simulink model "gm_Watermarker_ref"  (R2022a)
settings: Solver=FixedStepDiscrete  StartTime=0.0  StopTime=256*256-1  RelTol=1e-3
libraries: hdlsllib x10, dspsrcs4 x4
Description:
  | Performs watermarking.
  | In:
  | - One channel of 8-bit image 256x256
  | - Watermark (64 bits)
  | Out:
  | - Watermarked image channel
settings Model: SimulationMode=accelerator  Creator=The MathWorks, Inc.  LastModifiedBy=Администратор
settings SolverCC: AlgebraicLoopSolver=TrustRegion
settings DataIOCC: ExternalInput=image_and_mes_t.getElement('pixel_in'),image_and_mes_t.getElement('mes_in')  LimitDataPoints=on  LoadExternalInput=on  SaveFormat=Structure  SaveTime=off  ReturnWorkspaceOutputs=off
settings OptimizationCC: BlockReduction=off  ConditionallyExecuteInputs=off  DefaultParameterBehavior=Inlined  InheritOutputTypeSmallerThanSingle=on  OptimizeBlockIOStorage=off  DenormalBehavior=FlushToZero
settings DebuggingCC: AlgebraicLoopMsg=error  UnderspecifiedInitializationDetection=Classic  MergeDetectMultiDrivingBlocksExec=none  SolverPrmCheckMsg=warning  InheritedTsInSrcMsg=none  SingleTaskRateTransMsg=error  ParameterPrecisionLossMsg=none  UnconnectedInputMsg=warning  UnconnectedOutputMsg=warning  UnconnectedLineMsg=warning  AllowSymbolicDim=off  SFUnexpectedBacktrackingDiag=warning  SFNoUnconditionalDefaultTransitionDiag=warning  SFExecutionAtInitializationDiag=none  SFMachineParentedDataDiag=warning  ArithmeticOperatorsInVariantConditions=warning
settings HardwareCC: ProdBitPerPointer=32  ProdBitPerSizeT=32  ProdBitPerPtrDiffT=32  ProdLargestAtomicFloat=None  ProdIntDivRoundTo=Undefined  ProdEndianess=Unspecified  ProdWordSize=32  ProdHWDeviceType=ASIC/FPGA->ASIC/FPGA  TargetBitPerPointer=64  TargetBitPerSizeT=64  TargetBitPerPtrDiffT=64  TargetLongLongMode=on  TargetIntDivRoundTo=Zero  TargetEndianess=LittleEndian  TargetWordSize=64  TargetHWDeviceType=Generic->Custom  ProdEqTarget=off
settings ModelReferenceCC: PropagateSignalLabelsOutOfModel=off
settings SFSimCC: SimUseLocalCustomCode=off  CustomCodeUndefinedFunction=UseInterfaceOnly
settings RTWCC: Description=SystemVerilog DPI Component Generator  SystemTargetFile=systemverilog_dpi_grt.tlc  TemplateMakefile=systemverilog_dpi_grt_default_tmf  RTWVerbose=off  RTWUseLocalCustomCode=off  BuildConfiguration=Faster Runs  DLArmComputeVersion=19.05
settings CodeAppCC: MaxIdLength=256  StateflowObjectComments=on
settings DPIGRTTargetCC: TargetFcnLib=ansi_tfl_table_tmw.mat  GenFloatMathFcnCalls=NOT IN USE  TargetLangStandard=C89/C90 (ANSI)  CodeReplacementLibrary=None  UtilityFuncGeneration=Auto  MultiwordTypeDef=System defined  MultiwordLength=2048  DynamicStringBufferSize=256  GenerateFullHeader=on  InferredTypesCompatibility=off  GenerateSampleERTMain=off  GenerateTestInterfaces=off  ModelReferenceCompliant=on  ParMdlRefBuildCompliant=on  CompOptLevelCompliant=off  ConcurrentExecutionCompliant=off  IncludeMdlTerminateFcn=on  CombineOutputUpdateFcns=off  CombineSignalStateStructs=on  GroupInternalDataByFunction=off  SuppressErrorStatus=off  IncludeFileDelimiter=Auto  ERTCustomFileBanners=off  SupportAbsoluteTime=on  LogVarNameModifier=rt_  MatFileLogging=off  CodeInterfacePackaging=Reusable function  PurelyIntegerCode=off  SupportNonFinite=on  SupportComplex=on  SupportContinuousTime=on  SupportNonInlinedSFcns=on  RemoveDisableFunc=off  RemoveResetFunc=off  SupportVariableSizeSignals=off  ParenthesesLevel=Nominal  CastingMode=Nominal  MATLABClassNameForMDSCustomization=Simulink.SoftwareTarget.TargetSpecificTriggerConfigurationBase  ModelStepFunctionPrototypeControlCompliant=off  CPPClassGenCompliant=off  AutosarCompliant=off  MDXCompliant=off  GRTInterface=off  GenerateAllocFcn=on  UseToolchainInfoCompliant=on  GenerateSharedConstants=on  CoderGroups=[]  AccessMethods=[]  LookupTableObjectStructAxisOrder=1,2,3,4,...  LUTObjectStructOrderExplicitValues=Size,Breakpoints,Table  LUTObjectStructOrderEvenSpacing=Size,Breakpoints,Table  ArrayLayout=Column-major  UnsupportedSFcnMsg=error  ERTHeaderFileRootName=$R$E  ERTSourceFileRootName=$R$E  ERTDataFileRootName=$R_data  OptimizeReductions=off  RTWCAPISignals=on  RTWCAPIParams=off  RTWCAPIStates=off  RTWCAPIRootIO=off  ExtMode=off  ExtModeTransport=0  ExtModeStaticAlloc=off  ExtModeStaticAllocSize=1000000  ExtModeTesting=off  ExtModeMexFile=ext_comm  GenerateASAP2=off  MultiInstanceErrorCode=Error  DPICustomizeSystemVerilogCode=on  DPISystemVerilogTemplate=hdlverifier_dpitb_template.vgt  DPIReportRunTimeError=off  DPIRunTimeErrorSeverity=Fatal  DPIScalarizePorts=off  DPIGenerateTestBench=off  DPITestBenchSimulator=Mentor Graphics Questasim  DPITestPointAccessFcnInterface=None  DPIFixedPointDataType=CompatibleCType  DPIPortConnection=Port list  DPICompositeDataType=Flattened  DPIComponentTemplateType=Sequential
settings ConfigComp: CovMetricSettings=dw  CovSaveCumulativeToWorkspaceVar=on  CovSaveSingleToWorkspaceVar=on  CovExternalEMLEnable=off  CovSFcnEnable=off

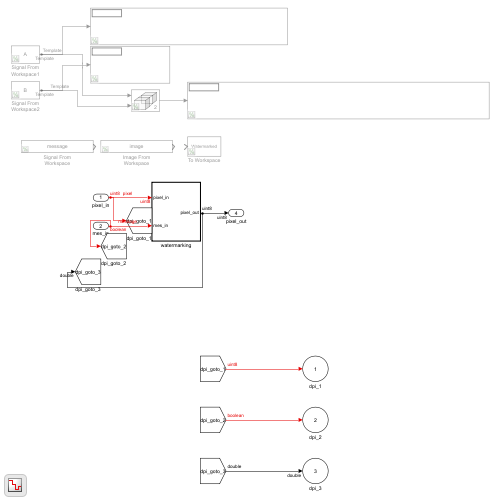
[thumbnail: Simulink's stored preview of the top-level diagram]
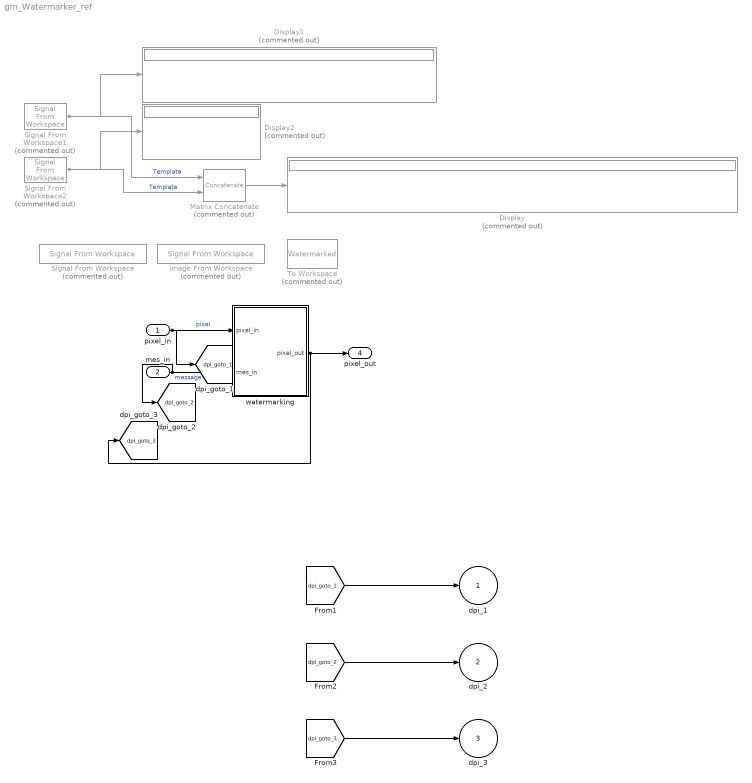
== system gm_Watermarker_ref ==
  pixel_in : Inport  OutDataTypeStr=uint8
  mes_in : Inport  Port=2  OutDataTypeStr=boolean
  Display : Display  Commented=on
      settings: Format=binary (Stored Integer)  Decimation=2
  Display1 : Display  Commented=on
      settings: Format=binary (Stored Integer)
  Display2 : Display  Commented=on
      settings: Format=binary (Stored Integer)
  Image From Workspace : dspsrcs4/Signal From Workspace  Commented=on  X=image  Ts=1  nsamps=1  OutputAfterFinalValue=Cyclic repetition  ignoreOrWarnInputAndFrameLengths=off  OutputFrames=off
  Matrix Concatenate : Concatenate  Commented=on  Mode=Multidimensional array  ConcatenateDimension=2
  Signal From Workspace : dspsrcs4/Signal From Workspace  Commented=on  X=message  Ts=1  nsamps=1  OutputAfterFinalValue=Cyclic repetition  ignoreOrWarnInputAndFrameLengths=off  OutputFrames=off
  Signal From Workspace1 : dspsrcs4/Signal From Workspace  Commented=on  X=A  Ts=1  nsamps=1  OutputAfterFinalValue=Cyclic repetition  ignoreOrWarnInputAndFrameLengths=off  OutputFrames=off
  Signal From Workspace2 : dspsrcs4/Signal From Workspace  Commented=on  X=B  Ts=1  nsamps=1  OutputAfterFinalValue=Cyclic repetition  ignoreOrWarnInputAndFrameLengths=off  OutputFrames=off
  To Workspace : ToWorkspace  Commented=on  VariableName=Watermarked  SampleTime=-1
      settings: Save2DSignal=2-D array (concatenate along first dimension)
  watermarking : Subsystem  TreatAsAtomicUnit=on
  dpi_1 : Outport
  dpi_2 : Outport  Port=2
  dpi_3 : Outport  Port=3
  pixel_out : Outport  Port=4  OutDataTypeStr=uint8
  tag scope: dpi_goto_1=global, dpi_goto_2=global, dpi_goto_3=global
  wires:
  pixel_in/1 -> watermarking/1(pixel_in), [dpi_goto_1]  "pixel"
  mes_in/1 -> watermarking/2(mes_in), [dpi_goto_2]  "message"
  Signal From Workspace1/1 -> Display1/1, Matrix Concatenate/1  "Template"
  Signal From Workspace2/1 -> Matrix Concatenate/2, Display2/1  "Template"
  Matrix Concatenate/1 -> Display/1
  watermarking/1(pixel_out) -> pixel_out/1, [dpi_goto_3]
  [dpi_goto_1] -> dpi_1/1
  [dpi_goto_2] -> dpi_2/1
  [dpi_goto_3] -> dpi_3/1

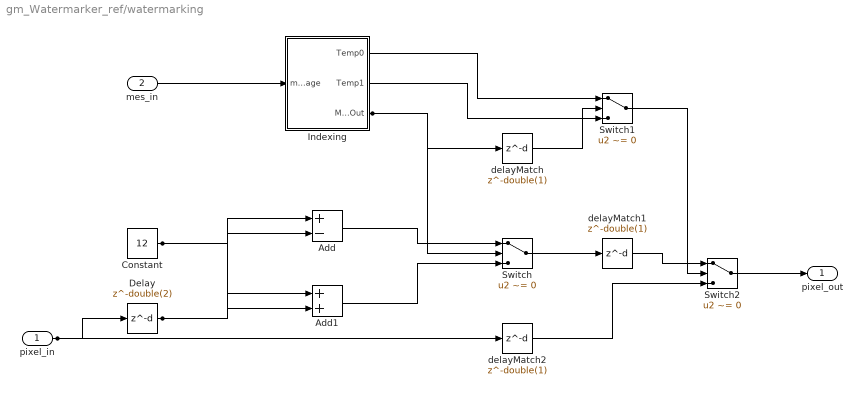
== system gm_Watermarker_ref/watermarking ==
  pixel_in : Inport  OutDataTypeStr=uint8  PortDimensions=1  SampleTime=1
  mes_in : Inport  Port=2  OutDataTypeStr=boolean  PortDimensions=1  SampleTime=1
  Add : Sum  Inputs=+-  AccumDataTypeStr=uint8  OutDataTypeStr=uint8  SampleTime=1
  Add1 : Sum  AccumDataTypeStr=uint8  OutDataTypeStr=uint8  SampleTime=1
  Constant : Constant  Value=12  OutDataTypeStr=uint8  SampleTime=1
  Delay : Delay  DelayLength=double(2)  InitialCondition=0  SampleTime=1
  Indexing : Subsystem
  Switch : Switch  Criteria=u2 ~= 0  Threshold=double(0)  OutDataTypeStr=uint8  SampleTime=1  SaturateOnIntegerOverflow=off  InputSameDT=off
  Switch1 : Switch  Criteria=u2 ~= 0  Threshold=double(0)  OutDataTypeStr=boolean  SampleTime=1  SaturateOnIntegerOverflow=off  InputSameDT=off
  Switch2 : Switch  Criteria=u2 ~= 0  Threshold=double(0)  OutDataTypeStr=uint8  SampleTime=1  SaturateOnIntegerOverflow=off  InputSameDT=off
  delayMatch : Delay  DelayLength=double(1)  InitialCondition=0  SampleTime=1
  delayMatch1 : Delay  DelayLength=double(1)  InitialCondition=0  SampleTime=1
  delayMatch2 : Delay  DelayLength=double(1)  InitialCondition=0  SampleTime=1
  pixel_out : Outport  SampleTime=1  VectorParamsAs1DForOutWhenUnconnected=off
  wires:
  pixel_in/1 -> Delay/1, delayMatch2/1
  Switch/1 -> delayMatch1/1
  Indexing/3(MessageOut) -> Switch/2, delayMatch/1
  Switch2/1 -> pixel_out/1
  Switch1/1 -> Switch2/2
  delayMatch1/1 -> Switch2/1
  delayMatch/1 -> Switch1/2
  Indexing/2(Temp1) -> Switch1/3
  Indexing/1(Temp0) -> Switch1/1
  Delay/1 -> Add/1, Add1/2
  Constant/1 -> Add/2, Add1/1
  Add1/1 -> Switch/3
  Add/1 -> Switch/1
  mes_in/1 -> Indexing/1(message)
  delayMatch2/1 -> Switch2/3

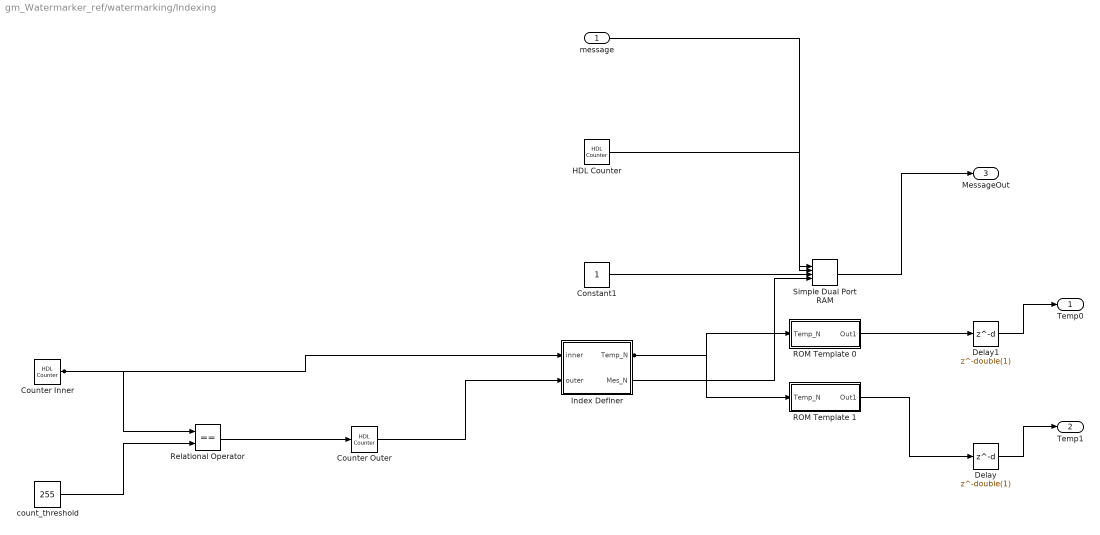
== system gm_Watermarker_ref/watermarking/Indexing ==
  message : Inport  OutDataTypeStr=boolean  PortDimensions=1  SampleTime=1
  Constant1 : Constant  OutDataTypeStr=boolean  SampleTime=1
  Counter Inner : hdlsllib/Sources/HDL Counter  CountType=Count limited  CountInit=0  CountStep=1  CountMax=255  CountFromType=Initial value  CountFrom=0  CountResetPort=off  CountLoadPort=off  CountEnbPort=off  CountDirPort=off  CountHitOutputPort=off  CountDataType=Unsigned  CountWordLen=8  CountFracLen=0  CountSampTime=1
  Counter Outer : hdlsllib/Sources/HDL Counter  CountType=Count limited  CountInit=0  CountStep=1  CountMax=255  CountFromType=Initial value  CountFrom=0  CountResetPort=off  CountLoadPort=off  CountEnbPort=on  CountDirPort=off  CountHitOutputPort=off  CountDataType=Unsigned  CountWordLen=8  CountFracLen=0  CountSampTime=1
  Delay : Delay  DelayLength=double(1)  InitialCondition=0  SampleTime=1
  Delay1 : Delay  DelayLength=double(1)  InitialCondition=0  SampleTime=1
  HDL Counter : hdlsllib/Sources/HDL Counter  CountType=Count limited  CountInit=0  CountStep=1  CountMax=63  CountFromType=Initial value  CountFrom=0  CountResetPort=off  CountLoadPort=off  CountEnbPort=off  CountDirPort=off  CountHitOutputPort=off  CountDataType=Unsigned  CountWordLen=6  CountFracLen=0  CountSampTime=1
  Index Definer : Subsystem
  ROM Template 0 : Subsystem
  ROM Template 1 : Subsystem
  Relational Operator : RelationalOperator  Operator===  OutDataTypeStr=boolean  SampleTime=1  InputSameDT=off
  Simple Dual Port RAM : hdlsllib/HDL RAMs/Simple Dual Port RAM  ram_size=6
      settings: SourceProductBaseCode=SL
  count_threshold : Constant  Value=255  OutDataTypeStr=uint8  SampleTime=1
  Temp0 : Outport  SampleTime=1
  Temp1 : Outport  Port=2  SampleTime=1
  MessageOut : Outport  Port=3  SampleTime=1
  wires:
  message/1 -> Simple Dual Port RAM/1
  count_threshold/1 -> Relational Operator/2
  Simple Dual Port RAM/1 -> MessageOut/1
  Relational Operator/1 -> Counter Outer/1
  ROM Template 1/1(Out1) -> Delay/1
  ROM Template 0/1(Out1) -> Delay1/1
  Index Definer/2(Mes_N) -> Simple Dual Port RAM/4
  Index Definer/1(Temp_N) -> ROM Template 1/1(Temp_N), ROM Template 0/1(Temp_N)
  HDL Counter/1 -> Simple Dual Port RAM/2
  Delay1/1 -> Temp0/1
  Delay/1 -> Temp1/1
  Counter Outer/1 -> Index Definer/2(outer)
  Counter Inner/1 -> Index Definer/1(inner), Relational Operator/1
  Constant1/1 -> Simple Dual Port RAM/3

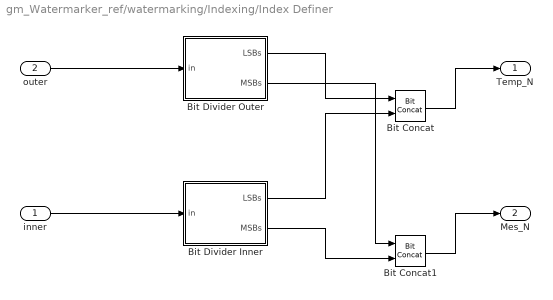
== system gm_Watermarker_ref/watermarking/Indexing/Index Definer ==
  inner : Inport  OutDataTypeStr=uint8  PortDimensions=1  SampleTime=1
  outer : Inport  Port=2  OutDataTypeStr=uint8  PortDimensions=1  SampleTime=1
  Bit Concat : hdlsllib/Logic and Bit Operations/Bit Concat  numInputs=2
  Bit Concat1 : hdlsllib/Logic and Bit Operations/Bit Concat  numInputs=2
  Bit Divider Inner : Subsystem
  Bit Divider Outer : Subsystem
  Temp_N : Outport  SampleTime=1
  Mes_N : Outport  Port=2  SampleTime=1
  wires:
  outer/1 -> Bit Divider Outer/1(in)
  inner/1 -> Bit Divider Inner/1(in)
  Bit Divider Outer/2(MSBs) -> Bit Concat1/1
  Bit Divider Outer/1(LSBs) -> Bit Concat/1
  Bit Divider Inner/2(MSBs) -> Bit Concat1/2
  Bit Divider Inner/1(LSBs) -> Bit Concat/2
  Bit Concat1/1 -> Mes_N/1
  Bit Concat/1 -> Temp_N/1

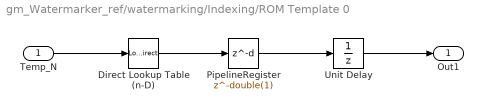
== system gm_Watermarker_ref/watermarking/Indexing/ROM Template 0 ==
  Temp_N : Inport  OutDataTypeStr=fixdt(0, 10, 0)  PortDimensions=1  SampleTime=1
  Direct Lookup Table (n-D) : LookupNDDirect  NumberOfTableDimensions=1  Table="reshape(logical([1 1 1 0 0 0 0 0 1 1 1 0 0 0 0 0 0 0 0 0 0 1 1 1 0 0 0 0 0 1 1 1 1 1 0 0 0 0 0 0 0 0 1 1 1 0 0 0 0 0 0 0 1 1 0 0 0 0 0 0 0 0 0 1 0 0 0 0 0 0 0 0 0 0 0 1 1 1 0 0 0 0 1 1 1 0 0 0 0 0 0 0 0 0 0 0 0 0 0 0 0 0 0 0 0 0 0 0 0 1 1 1 1 1 1 1 0 0 0 0 0 0 0 0 0 0 0 0 0 0 0 0 0 0 0 0 0 0 0 0 0 0 1 1 1 1 0 0 0 0 0 0 0 0 0 0 0 0 0 0 0 0 0 0 0 0 0 0 0 0 0 0 0 0 0 0 0 0 0 0 0 0 0 0 0 0 0 0 0 0 0 0 0 0 0 1 1 1 1 1 1 0 0 0 0 0 0 0 0 0 0 0 0 0 0 0 1 1 1 1 1 0 0 0 0 1 1 1 1 1 1 1 1 1 0 0 0 0 0 0 0 0 0 0 0 0 1 1 1 1 1 1 1 1 1 0 1 1 1 0 0 0 0 0 0 1 1 0 0 0 0 0 0 0 0 0 0 1 1 1 0 0 0 0 0 1 1 1 1 0 0 0 0 0 0 0 0 0 1 1 1 0 0 0 0 0 0 0 1 1 0 0 0 0 0 0 0 0 0 1 0 0 0 0 0 0 0 0 0 0 0 1 1 1 0 0 0 0 1 1 1 0 0 0 0 0 0 0 0 0 0 0 0 0 0 0 0 0 0 0 0 0 0 0 0 1 1 1 1 1 1 1 0 0 0 0 0 0 0 0 0 0 0 0 0 0 0 0 0 0 0 0 0 0 0 0 0 0 1 1 1 1 0 0 0 0 0 0 0 0 0 0 0 0 0 0 0 0 0 0 0 1 1 1 0 0 0 0 0 0 0 0 0 0 0 0 0 0 0 0 0 0 1 1 1 0 0 0 0 0 0 1 1 1 1 1 1 0 0 0 0 0 0 0 0 0 0 0 0 0 0 0 1 1 1 1 1 1 0 0 0 1 1 1 1 0 1 1 1 1 0 0 0 0 0 0 0 0 0 0 0 0 1 1 1 1 0 1 1 1 1 0 1 1 1 0 0 0 0 0 0 1 1 0 0 0 0 0 0 0 0 0 0 1 1 1 0 0 0 0 0 1 1 1 1 0 0 0 0 0 0 0 0 0 1 1 1 0 0 0 0 0 0 1 1 1 0 0 0 0 0 0 0 0 0 1 0 0 0 0 0 0 0 0 0 0 0 1 1 1 0 0 0 0 1 1 1 0 0 0 0 0 0 0 0 0 0 0 0 0 0 0 0 0 0 0 0 0 0 0 0 1 1 1 1 1 1 0 0 0 0 0 0 0 0 0 0 0 0 0 0 0 0 0 0 0 0 0 0 0 0 0 0 0 1 1 1 1 0 0 0 0 0 0 0 0 0 0 0 0 0 0 0 0 0 0 0 1 1 1 0 0 0 0 0 0 0 0 0 0 0 0 0 0 0 0 0 1 1 1 0 0 0 0 0 0 0 1 1 1 1 1 1 0 0 0 0 0 0 0 0 0 0 0 0 0 0 0 1 1 1 1 1 1 0 0 0 1 1 1 1 0 1 1 1 1 0 0 0 0 0 0 0 0 0 0 0 0 1 1 1 1 0 1 1 1 1 0 1 1 1 0 0 0 0 0 0 1 1 0 0 0 0 0 0 0 0 0 0 1 1 1 0 0 0 0 0 0 1 1 1 0 0 0 0 0 0 0 0 0 1 1 1 0 0 0 0 0 0 1 1 1 0 0 0 0 0 0 0 0 0 1 0 0 0 0 0 0 0 0 0 0 0 1 1 1 1 0 0 0 1 1 1 0 0 0 0 0 0 0 0 0 0 0 0 0 0 0 0 0 0 0 0 0 0 0 0 1 1 1 1 1 1 1 0 0 0 0 0 0 0 0 0 0 0 0 0 0 0 0 0 0 0 0 0 0 0 0 0 0 1 1 1 1 0 0 0 0 0 0 0 0 0 0 0 0 0 0 0 0 0 0 0 1 1 0 0 0 0 0 0 0 0 0 0 0 0 0 0 0 0 0 0 0 1 1 0 0 0 0 0 0 0 1 1 1 1 1 1 0 0 0 0 0 0 0 0 0 0 0 0 0 0 1 1 1 1 1 1 1 0 0 0 1 1 1 1 0 1 1 1 1 0 0 0 0 0 0 0 0 0 0 0 0 1 1 1 1 0 0 1 1 1 0]).', [1024     1])"  DiagnosticForOutOfRangeInput=Error  SampleTime=1  TableDataTypeStr=boolean
  PipelineRegister : Delay  DelayLength=double(1)  InitialCondition=0  SampleTime=1
  Unit Delay : UnitDelay  SampleTime=1
  Out1 : Outport  SampleTime=1
  wires:
  Direct Lookup Table (n-D)/1 -> PipelineRegister/1
  Temp_N/1 -> Direct Lookup Table (n-D)/1
  Unit Delay/1 -> Out1/1
  PipelineRegister/1 -> Unit Delay/1

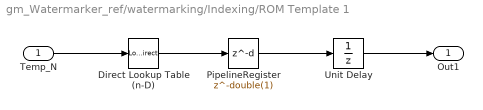
== system gm_Watermarker_ref/watermarking/Indexing/ROM Template 1 ==
  Temp_N : Inport  OutDataTypeStr=fixdt(0, 10, 0)  PortDimensions=1  SampleTime=1
  Direct Lookup Table (n-D) : LookupNDDirect  NumberOfTableDimensions=1  Table="reshape(logical([1 1 0 0 0 0 0 0 0 0 0 1 1 1 0 0 0 0 0 0 1 1 0 0 0 0 0 0 0 0 0 0 1 1 1 0 0 0 0 0 0 0 1 1 1 0 0 0 0 0 0 0 0 1 1 1 0 0 0 0 0 0 0 1 0 1 1 1 1 0 0 0 1 1 1 0 0 0 0 0 0 0 0 0 0 0 1 1 1 1 0 0 0 1 1 1 0 0 0 1 1 1 1 1 1 1 0 0 0 0 0 0 0 0 0 0 0 0 0 0 1 1 1 1 1 1 1 0 0 0 0 0 0 1 1 1 0 0 0 0 0 0 0 0 0 0 0 0 0 0 0 0 0 0 1 1 1 0 0 0 0 0 0 0 0 0 0 0 0 0 0 0 0 0 0 0 1 1 0 0 0 0 0 0 0 0 0 0 0 0 0 0 0 0 0 0 0 0 0 0 0 0 0 0 0 0 1 1 1 1 1 1 0 0 0 0 0 0 0 0 0 0 0 0 0 0 0 0 0 0 0 0 0 0 0 0 1 1 1 1 1 1 1 1 1 0 0 0 0 0 0 0 0 0 0 0 1 1 0 0 0 0 0 0 0 0 0 1 1 1 1 0 0 0 0 1 1 1 0 0 0 0 0 0 0 0 0 0 1 1 1 0 0 0 0 0 0 0 1 1 1 0 0 0 0 0 0 0 0 1 1 1 0 0 0 0 0 0 0 1 0 1 1 1 1 0 0 0 1 1 1 0 0 0 0 0 0 0 0 0 0 0 1 1 1 1 0 0 0 1 1 1 0 0 0 1 1 1 1 1 1 1 0 0 0 0 0 0 0 0 0 0 0 0 0 0 1 1 1 1 1 1 1 0 0 0 0 0 0 1 1 1 0 0 0 0 0 0 0 0 0 0 0 0 0 0 0 0 0 1 1 1 1 0 0 0 0 0 0 0 0 0 0 0 0 0 0 0 0 0 0 0 1 1 0 0 0 0 0 0 0 0 0 0 0 0 0 0 0 0 0 0 0 0 0 0 0 0 0 0 0 0 1 1 1 1 1 1 0 0 0 0 0 0 0 0 0 0 0 0 0 0 0 0 0 0 0 0 0 0 0 0 1 1 1 1 1 1 1 1 1 0 0 0 0 0 0 0 0 0 0 0 1 1 0 0 0 0 0 0 0 0 0 1 1 1 1 0 0 0 0 1 1 1 0 0 0 0 0 0 0 0 0 0 1 1 1 0 0 0 0 0 0 0 1 1 0 0 0 0 0 0 0 0 0 1 1 1 0 0 0 0 0 0 0 1 0 0 1 1 1 0 0 0 1 1 1 0 0 0 0 0 0 0 0 0 0 0 1 1 1 1 0 0 0 1 1 1 0 0 0 1 1 1 1 1 1 1 0 0 0 0 0 0 0 0 0 0 0 0 0 0 1 1 1 1 1 1 1 0 0 0 0 0 0 1 1 1 0 0 0 0 0 0 0 0 0 0 0 0 0 0 0 0 0 0 1 1 1 0 0 0 0 0 0 0 0 0 0 0 0 0 0 0 0 0 0 0 1 1 0 0 0 0 0 0 0 0 0 0 0 0 0 0 0 0 0 0 0 0 0 0 0 0 0 0 0 0 1 1 1 1 1 1 0 0 0 0 0 0 0 0 0 0 0 0 0 0 0 0 0 0 0 0 0 0 0 0 1 1 1 1 1 1 1 1 1 0 0 0 0 0 0 0 0 0 0 0 1 1 0 0 0 0 0 0 0 0 0 1 1 1 1 0 0 0 0 1 1 1 1 0 0 0 0 0 0 0 0 0 1 1 1 0 0 0 0 0 0 0 1 1 0 0 0 0 0 0 0 0 0 1 1 1 0 0 0 0 0 0 0 1 0 0 1 1 1 0 0 0 1 1 1 0 0 0 0 0 0 0 0 0 0 0 0 1 1 1 0 0 0 1 1 1 0 0 0 1 1 1 1 1 1 1 0 0 0 0 0 0 0 0 0 0 0 0 0 0 1 1 1 1 1 1 1 0 0 0 0 0 0 1 1 1 0 0 0 0 0 0 0 0 0 0 0 0 0 0 0 0 0 0 1 1 1 0 0 0 0 0 0 0 0 0 0 0 0 0 0 0 0 0 0 0 0 0 0 0 0 0 0 0 0 0 0 0 0 0 0 0 0 0 0 0 0 0 0 0 0 0 0 0 0 0 1 1 1 1 1 1 0 0 0 0 0 0 0 0 0 0 0 0 0 0 0 0 0 0 0 0 0 0 0 0 1 1 1 1 0 1 1 1 1 0 0 0 0 0 0 0 0 0 0 0]).', [1024     1])"  DiagnosticForOutOfRangeInput=Error  SampleTime=1  TableDataTypeStr=boolean
  PipelineRegister : Delay  DelayLength=double(1)  InitialCondition=0  SampleTime=1
  Unit Delay : UnitDelay  SampleTime=1
  Out1 : Outport  SampleTime=1
  wires:
  Direct Lookup Table (n-D)/1 -> PipelineRegister/1
  Temp_N/1 -> Direct Lookup Table (n-D)/1
  Unit Delay/1 -> Out1/1
  PipelineRegister/1 -> Unit Delay/1

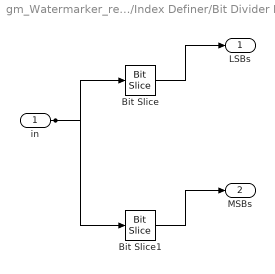
== system gm_Watermarker_ref/watermarking/Indexing/Index Definer/Bit Divider Inner ==
  in : Inport  OutDataTypeStr=uint8  PortDimensions=1  SampleTime=1
  Bit Slice : hdlsllib/Logic and Bit Operations/Bit Slice  lidx=double(4)  ridx=double(0)
      settings: SourceProductBaseCode=SL
  Bit Slice1 : hdlsllib/Logic and Bit Operations/Bit Slice  lidx=double(7)  ridx=double(5)
      settings: SourceProductBaseCode=SL
  LSBs : Outport  SampleTime=1
  MSBs : Outport  Port=2  SampleTime=1
  wires:
  in/1 -> Bit Slice/1, Bit Slice1/1
  Bit Slice1/1 -> MSBs/1
  Bit Slice/1 -> LSBs/1

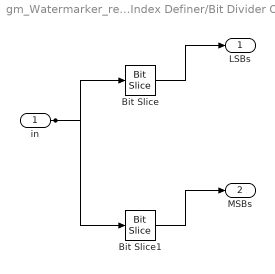
== system gm_Watermarker_ref/watermarking/Indexing/Index Definer/Bit Divider Outer ==
  in : Inport  OutDataTypeStr=uint8  PortDimensions=1  SampleTime=1
  Bit Slice : hdlsllib/Logic and Bit Operations/Bit Slice  lidx=double(4)  ridx=double(0)
      settings: SourceProductBaseCode=SL
  Bit Slice1 : hdlsllib/Logic and Bit Operations/Bit Slice  lidx=double(7)  ridx=double(5)
      settings: SourceProductBaseCode=SL
  LSBs : Outport  SampleTime=1
  MSBs : Outport  Port=2  SampleTime=1
  wires:
  in/1 -> Bit Slice/1, Bit Slice1/1
  Bit Slice1/1 -> MSBs/1
  Bit Slice/1 -> LSBs/1
